simulink model "comprehensive_model_with_rocks_trial"  (R2019a)
settings: Solver=FixedStepAuto  StartTime=0.0  StopTime=15  FixedStep=0.001  RelTol=1e-3
PreLoadFcn:
  | load('tumbleweed_constants.mat')
values from neighbouring files (symbols this model uses):
  Ar = 0.785398163397    [tumbleweed_constants.mat]
  CD = 0.8    [tumbleweed_constants.mat]
  d = 0.65    [tumbleweed_constants.mat]
  g = 9.81    [tumbleweed_constants.mat]
  Ixx = 1.29    [tumbleweed_constants.mat]
  Iyy = 1.29    [tumbleweed_constants.mat]
  Izz = 1.29    [tumbleweed_constants.mat]
  m = 1    [tumbleweed_constants.mat]
  maxr = 0.45    [tumbleweed_constants.mat]
  mf = 14    [tumbleweed_constants.mat]
  minr = 0.2    [tumbleweed_constants.mat]
  mu0 = 0.02    [tumbleweed_constants.mat]
  muk = 0.5    [tumbleweed_constants.mat]
  must = 0.8    [tumbleweed_constants.mat]
  R = cylR*ones(size(Theta,1),size(Theta,2))    [d3_animate.m]    (also in tumbleweed_constants.mat = 0.5)
  rest_coeff = 0.6    [tumbleweed_constants.mat]
  rho = 1.2    [tumbleweed_constants.mat]
  ts = 0.5    [tumbleweed_constants.mat]
  v_thres = 0.0001    [tumbleweed_constants.mat]
  vmax = 0.2    [tumbleweed_constants.mat]
  YY = 50    [tumbleweed_constants.mat]
libraries: simulink x2
(part 2 of 9)

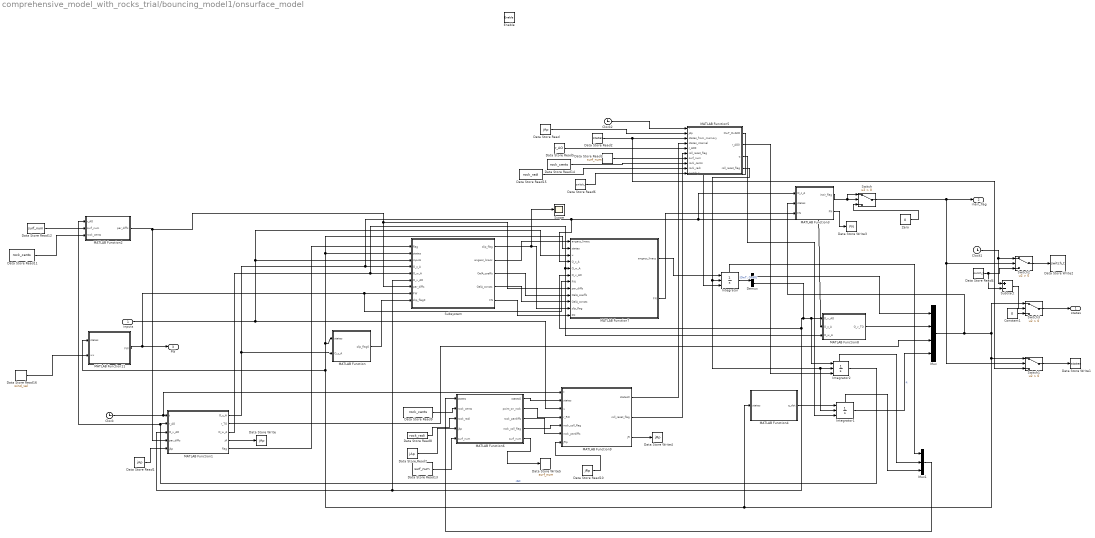
== system comprehensive_model_with_rocks_trial/bouncing_model1/onsurface_model ==
  "inputs " : Inport
  Enable : EnablePort  StatesWhenEnabling=reset
  Clock : Clock
  Clock1 : Clock
  Clock2 : Clock
  Constant1 : Constant  Value=0  VectorParams1D=off
  Data Store Read : DataStoreRead  DataStoreName=jAp
  Data Store Read1 : DataStoreRead  DataStoreName=jAp
  Data Store Read10 : DataStoreRead  DataStoreName=jRp
  Data Store Read11 : DataStoreRead  DataStoreName=rock_cents
  Data Store Read12 : DataStoreRead  DataStoreName=surf_num
  Data Store Read13 : DataStoreRead  DataStoreName=surf_num
  Data Store Read14 : DataStoreRead  DataStoreName=rock_cents
  Data Store Read15 : DataStoreRead  DataStoreName=rock_radi
  Data Store Read16 : DataStoreRead  DataStoreName=wind_vel
  Data Store Read2 : DataStoreRead  DataStoreName=states
  Data Store Read3 : DataStoreRead  DataStoreName=surf_num
  Data Store Read4 : DataStoreRead  DataStoreName=switch_t
  Data Store Read5 : DataStoreRead  DataStoreName=r_AO
  Data Store Read6 : DataStoreRead  DataStoreName=switch_t
  Data Store Read7 : DataStoreRead  DataStoreName=jAp
  Data Store Read8 : DataStoreRead  DataStoreName=rock_radi
  Data Store Read9 : DataStoreRead  DataStoreName=rock_cents
  Data Store Write : DataStoreWrite  DataStoreName=jAp
  Data Store Write1 : DataStoreWrite  DataStoreName=states
  Data Store Write2 : DataStoreWrite  DataStoreName=switch_t
  Data Store Write3 : DataStoreWrite  DataStoreName=FN
  Data Store Write4 : DataStoreWrite  DataStoreName=jRp
  Data Store Write5 : DataStoreWrite  DataStoreName=surf_num
  Demux : Demux  Outputs=[3;3]
  Integrator : Integrator  ExternalReset=level hold  InitialConditionSource=external  ShowStatePort=on
  Integrator1 : Integrator  ExternalReset=level hold  InitialConditionSource=external  ShowStatePort=on
  Integrator2 : Integrator  ExternalReset=level hold  InitialConditionSource=external  InitialCondition=[0;0;10]  ShowStatePort=on
  MATLAB Function : MATLAB Function  TreatAsAtomicUnit=on
  MATLAB Function1 : MATLAB Function  Priority=1  TreatAsAtomicUnit=on
  MATLAB Function11 : MATLAB Function  TreatAsAtomicUnit=on
  MATLAB Function2 : MATLAB Function  TreatAsAtomicUnit=on
  MATLAB Function3 : MATLAB Function  TreatAsAtomicUnit=on
  MATLAB Function4 : MATLAB Function  TreatAsAtomicUnit=on
  MATLAB Function5 : MATLAB Function  TreatAsAtomicUnit=on
  MATLAB Function6 : MATLAB Function  TreatAsAtomicUnit=on
  MATLAB Function7 : MATLAB Function  TreatAsAtomicUnit=on
  MATLAB Function8 : MATLAB Function  TreatAsAtomicUnit=on
  MATLAB Function9 : MATLAB Function  TreatAsAtomicUnit=on
  Mux : Mux  Inputs=[3;3;3;4]
  Mux1 : Mux  Inputs=[6;3;4]
  Scope : Scope
  Subsystem : Subsystem
  Subtract : Sum  Inputs=+-
  Switch{,1..3} (4 alike) : Switch  Criteria=u2 > Threshold
  Zero : Constant  Value=0  OutDataTypeStr=Inherit: Inherit via back propagation
  states : Outport
  inair_flag : Outport  Port=2  InitialOutput=1
  FW : Outport  Port=3
  wires:
  MATLAB Function2/1(par_diffs) -> MATLAB Function1/4(par_diffs), MATLAB Function7/8(par_diffs), Subsystem/7(par_diffs)
  MATLAB Function5/1(OwT_OvAO0) -> Integrator/3
  Subsystem/4(OalA_consts) -> MATLAB Function7/10(OalA_consts)
  Subsystem/3(OalA_coeffs) -> MATLAB Function7/9(OalA_coeffs)
  Subsystem/1(slip_flag) -> Scope/1, MATLAB Function7/11(slip_flag)
  Subsystem/2(angacc_linacc) -> MATLAB Function7/1("angacc_linacc ")
  MATLAB Function/1(slip_flag0) -> Subsystem/9(slip_flag0)
  "inputs "/1 -> MATLAB Function9/3(u), Subsystem/3(inputs), MATLAB Function7/3(u)
  MATLAB Function7/1(angacc_linacc) -> Integrator/1
  MATLAB Function1/5(flag) -> Subsystem/1(flag)
  Demux/2 -> Subsystem/6(O_v_AO), MATLAB Function1/3(O_v_AO), MATLAB Function7/6(O_v_AO), MATLAB Function8/1(O_v_AO), Integrator2/1
  Integrator/1 -> Demux/1  "[OwT; OvAO]"
  MATLAB Function4/1(q_dot) -> Integrator1/1
  MATLAB Function5/2(r_AO0) -> Integrator2/3
  MATLAB Function8/1(O_v_TO) -> Mux/2
  Demux/1 -> Mux/1
  Integrator2/1 -> MATLAB Function2/1(r_AO), MATLAB Function1/2(r_AO)  "rAO"
  MATLAB Function1/2(r_TO) -> Mux/3
  Integrator1/1 -> Mux/4  "q"
  MATLAB Function1/1(O_c_A) -> Subsystem/4(O_c_A), MATLAB Function8/2(O_c_A), MATLAB Function3/1(O_c_A), MATLAB Function7/4(O_c_A), MATLAB Function/2(O_c_A)
  MATLAB Function1/3(O_w_A) -> Subsystem/5(O_w_A), MATLAB Function8/3(O_w_A), MATLAB Function7/5(O_w_A)
  MATLAB Function11/1(FW) -> Subsystem/8(FW), MATLAB Function7/7(FW), FW/1
  Clock/1 -> MATLAB Function9/1(t), MATLAB Function1/1(t)
  Mux/1 -> MATLAB Function3/2(states), Subsystem/2(states), MATLAB Function7/2(states), MATLAB Function/1(states), MATLAB Function11/1(states), MATLAB Function4/1(states), Switch1/1, Switch3/1
  MATLAB Function1/4(jA) -> Data Store Write/1
  Data Store Read/1 -> MATLAB Function5/2(jAp)
  Data Store Read1/1 -> MATLAB Function1/5(jAp)
  Subsystem/5(FN) -> MATLAB Function7/12("FN ")
  MATLAB Function7/2(FN) -> MATLAB Function3/3("FN ")
  MATLAB Function3/1(inair_flag) -> Switch/1, Switch/2
  Switch/1 -> Switch2/2, Switch1/2, inair_flag/1
  Zero/1 -> Switch/3
  MATLAB Function5/3(q) -> Integrator1/3
  Switch1/1 -> Data Store Write1/1
  Switch2/1 -> Data Store Write2/1
  Data Store Read4/1 -> Subtract/2, Switch2/3
  Clock1/1 -> Subtract/1, Switch2/1
  Switch3/1 -> states/1
  Subtract/1 -> Switch3/2
  Constant1/1 -> Switch3/3
  Data Store Read5/1 -> MATLAB Function5/5("r_AO0 ")
  MATLAB Function3/2(FN) -> Data Store Write3/1
  MATLAB Function9/1(states0) -> MATLAB Function5/4(states_internal)
  Data Store Read2/1 -> Switch1/3, MATLAB Function5/3(states_from_memory)
  Data Store Read6/1 -> MATLAB Function5/10(switch_t)
  MATLAB Function6/4(rock_coll_flag) -> MATLAB Function9/5(rock_coll_flag)
  MATLAB Function6/3(rock_pardiffs) -> MATLAB Function9/6(rock_pardiffs)
  MATLAB Function6/2(point_on_rock) -> MATLAB Function9/4(r_RO)
  MATLAB Function6/1(states0) -> MATLAB Function9/2(states)
  Data Store Read7/1 -> MATLAB Function6/4(jAp)
  Data Store Read8/1 -> MATLAB Function6/3(rock_radi)
  Data Store Read9/1 -> MATLAB Function6/2(rock_cents)
  Mux1/1 -> MATLAB Function6/1(states)
  Integrator/State -> Mux1/1
  Integrator2/State -> Mux1/2
  Integrator1/State -> Mux1/3
  Data Store Read10/1 -> MATLAB Function9/7(jRp)
  MATLAB Function9/3(jR) -> Data Store Write4/1
  MATLAB Function9/2(roll_reset_flag) -> MATLAB Function5/6("roll_reset_flag ")
  MATLAB Function5/4(roll_reset_flag) -> Integrator/2, Integrator1/2, Integrator2/2
  Data Store Read3/1 -> MATLAB Function5/7(surf_num)
  Data Store Read11/1 -> MATLAB Function2/3(rock_cents)
  Data Store Read12/1 -> MATLAB Function2/2(surf_num)
  Data Store Read13/1 -> MATLAB Function6/5("surf_num ")
  Data Store Read14/1 -> MATLAB Function5/8(rock_cents)
  Data Store Read15/1 -> MATLAB Function5/9(rock_radi)
  Clock2/1 -> MATLAB Function5/1(t)
  MATLAB Function6/5(surf_num) -> Data Store Write5/1
  Data Store Read16/1 -> MATLAB Function11/2(wx)

== system comprehensive_model_with_rocks_trial/command filter based backstepper/Command filter ==
  alpha : Inport
  Demux : Demux  Commented=on  Outputs=3
  Demux1 : Demux  Commented=on  Outputs=2
  Demux2 : Demux  Commented=on  Outputs=2
  Demux3 : Demux  Commented=on  Outputs=2
  Demux4 : Demux  Outputs=3
  Gain : Gain  Gain=2
  Gain1 : Gain  Gain=2
  Gain2 : Gain  Gain=2
  Gain3 : Gain  Gain=5
  Gain4 : Gain  Gain=5
  Gain5 : Gain  Gain=5
  Integrator : Integrator
  Integrator1 : Integrator  InitialCondition=0.325
  Integrator2 : Integrator
  Integrator3 : Integrator
  Integrator4 : Integrator  InitialCondition=0.325
  Integrator5 : Integrator  InitialCondition=0.325
  Mux : Mux  Commented=on  Inputs=3
  Mux1 : Mux  Commented=on  Inputs=3
  Mux2 : Mux  Inputs=3
  Mux3 : Mux  Inputs=3
  State-Space : StateSpace  Commented=on  A=[0, 10; -2*0.8*10, -10]  B=[0;20]  C=[1,0;0,1]  D=[0;0]  InitialCondition=[0;0]
  State-Space1 : StateSpace  Commented=on  A=[0, 10; -2*0.8*10, -10]  B=[0;20]  C=[1,0;0,1]  D=[0;0]  InitialCondition=[0;0]
  State-Space2 : StateSpace  Commented=on  A=[0, 10; -2*0.8*10, -10]  B=[0;5]  C=[1,0;0,1]  D=[0;0]  InitialCondition=[0;0]
  Subtract{,1..5} (6 alike) : Sum  Inputs=+-
  wc : Outport
  wc_dot : Outport  Port=2
  wires:
  State-Space/1 -> Demux1/1
  Demux/1 -> State-Space/1
  Demux/2 -> State-Space1/1
  Demux/3 -> State-Space2/1
  State-Space1/1 -> Demux2/1
  Demux2/1 -> Mux/2
  State-Space2/1 -> Demux3/1
  Demux1/1 -> Mux/1
  Demux3/1 -> Mux/3
  Demux1/2 -> Mux1/1
  Demux2/2 -> Mux1/2
  Demux3/2 -> Mux1/3
  Mux2/1 -> wc/1
  alpha/1 -> Demux4/1
  Demux4/1 -> Subtract/1  "v1_sat"
  Gain3/1 -> Integrator/1
  Subtract/1 -> Gain/1  "v1_sat - z1"
  Subtract5/1 -> Gain5/1
  Gain/1 -> Subtract3/1
  Subtract2/1 -> Gain2/1
  Integrator2/1 -> Mux3/2, Subtract4/2, Integrator4/1
  Gain4/1 -> Integrator2/1
  Subtract1/1 -> Gain1/1
  Subtract3/1 -> Gain3/1
  Subtract4/1 -> Gain4/1
  Gain5/1 -> Integrator3/1
  Integrator/1 -> Integrator1/1, Mux3/1, Subtract3/2  "z2"
  Integrator5/1 -> Subtract2/2, Mux2/3
  Mux3/1 -> wc_dot/1
  Gain1/1 -> Subtract4/1
  Gain2/1 -> Subtract5/1
  Integrator4/1 -> Subtract1/2, Mux2/2
  Integrator3/1 -> Mux3/3, Subtract5/2, Integrator5/1
  Integrator1/1 -> Subtract/2, Mux2/1  "z1"
  Demux4/2 -> Subtract1/1
  Demux4/3 -> Subtract2/1

== system comprehensive_model_with_rocks_trial/command filter based backstepper/Subsystem ==
  v : Inport
  states : Inport  Port=2
  Add : Sum  Inputs=+-
  Add1 : Sum  Inputs=+-
  Add2 : Sum  Inputs=+-
  Demux : Demux  Outputs=3
  Derivative : Derivative  CoefficientInTFapproximation=0
  Gain : Gain  Gain=10^2
  Gain1 : Gain  Gain=2*0.1*10
  Gain2 : Gain  Gain=10^2
  Gain3 : Gain  Gain=2*0.1*10
  Gain4 : Gain  Gain=10^2
  Gain5 : Gain  Gain=2*0.1*10
  Integrator1 : Integrator  InitialCondition=d/2
  Integrator2 : Integrator  InitialCondition=d/2
  Integrator3 : Integrator  InitialCondition=d/2
  MATLAB Function : MATLAB Function  TreatAsAtomicUnit=on
  Mux : Mux  Inputs=3
  Mux1 : Mux  Inputs=3
  Saturation : Saturate  UpperLimit=vmax  LowerLimit=-vmax
  Saturation1 : Saturate  UpperLimit=vmax  LowerLimit=-vmax
  Saturation2 : Saturate  UpperLimit=maxr  LowerLimit=minr
  Saturation3 : Saturate  UpperLimit=maxr  LowerLimit=minr
  Saturation4 : Saturate  UpperLimit=vmax  LowerLimit=-vmax
  Saturation5 : Saturate  UpperLimit=maxr  LowerLimit=minr
  Subtract : Sum  Inputs=+-
  Subtract1 : Sum  Inputs=+-
  Subtract2 : Sum  Inputs=+-
  u : Outport
  u_dot : Outport  Port=2
  u_ddot : Outport  Port=3
  f3_u : Outport  Port=4
  wires:
  Saturation/1 -> Mux1/1, Gain1/1, Integrator1/1
  Demux/1 -> Saturation2/1
  Gain1/1 -> Subtract/2
  Gain/1 -> Subtract/1
  Subtract/1 -> Saturation/1
  Integrator1/1 -> Mux/1, Add/2
  Add/1 -> Gain/1
  Saturation2/1 -> Add/1
  v/1 -> Demux/1
  Saturation1/1 -> Integrator2/1, Mux1/2, Gain3/1
  Saturation3/1 -> Add1/1
  Add1/1 -> Gain2/1
  Integrator2/1 -> Add1/2, Mux/2
  Gain2/1 -> Subtract1/1
  Gain3/1 -> Subtract1/2
  Demux/2 -> Saturation3/1
  Subtract1/1 -> Saturation1/1
  Saturation4/1 -> Gain5/1, Integrator3/1
  Saturation5/1 -> Add2/1
  Add2/1 -> Gain4/1
  Integrator3/1 -> Mux1/3, Add2/2, Mux/3
  Gain4/1 -> Subtract2/1
  Gain5/1 -> Subtract2/2
  Demux/3 -> Saturation5/1
  Subtract2/1 -> Saturation4/1
  Mux1/1 -> Derivative/1, u_dot/1, MATLAB Function/2(u_dot)
  Mux/1 -> u/1, MATLAB Function/1(u)
  Derivative/1 -> MATLAB Function/3(u_ddot), u_ddot/1
  states/1 -> MATLAB Function/4(states)
  MATLAB Function/1(f3_u) -> f3_u/1

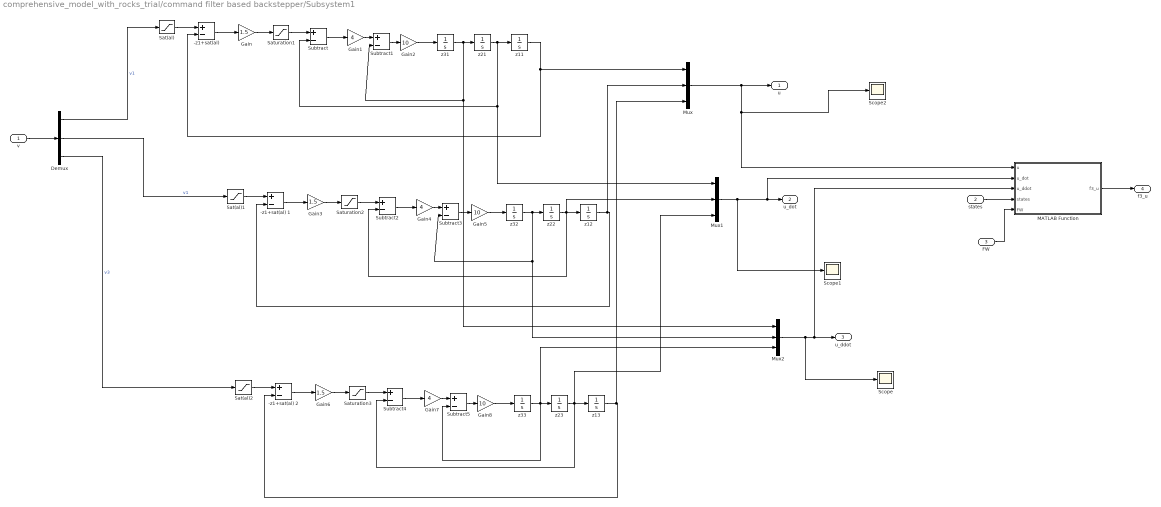
== system comprehensive_model_with_rocks_trial/command filter based backstepper/Subsystem1 ==
  v : Inport
  states : Inport  Port=2
  FW : Inport  Port=3
  "-z1+sat(al) " : Sum  Inputs=+-
  -z1+sat(al) 1 : Sum  Inputs=+-
  -z1+sat(al) 2 : Sum  Inputs=+-
  Demux : Demux  Outputs=3
  Gain : Gain  Gain=1.5
  Gain1 : Gain  Gain=4
  Gain2 : Gain  Gain=10
  Gain3 : Gain  Gain=1.5
  Gain4 : Gain  Gain=4
  Gain5 : Gain  Gain=10
  Gain6 : Gain  Gain=1.5
  Gain7 : Gain  Gain=4
  Gain8 : Gain  Gain=10
  MATLAB Function : MATLAB Function  TreatAsAtomicUnit=on
  Mux : Mux  Inputs=3
  Mux1 : Mux  Inputs=3
  Mux2 : Mux  Inputs=3
  Sat(al) : Saturate  UpperLimit=maxr  LowerLimit=minr  LinearizeAsGain=off
  Sat(al)1 : Saturate  UpperLimit=maxr  LowerLimit=minr  LinearizeAsGain=off
  Sat(al)2 : Saturate  UpperLimit=maxr  LowerLimit=minr
  Saturation1 : Saturate  UpperLimit=vmax  LowerLimit=-vmax
  Saturation2 : Saturate  UpperLimit=vmax  LowerLimit=-vmax
  Saturation3 : Saturate  UpperLimit=vmax  LowerLimit=-vmax
  Scope : Scope
  Scope1 : Scope
  Scope2 : Scope
  Subtract{,1..5} (6 alike) : Sum  Inputs=+-
  z11 : Integrator  InitialCondition=d/2
  z12 : Integrator  InitialCondition=d/2
  z13 : Integrator  InitialCondition=d/2
  z{21..23,31..33} (6 alike) : Integrator
  u : Outport
  u_dot : Outport  Port=2
  u_ddot : Outport  Port=3
  f3_u : Outport  Port=4
  wires:
  Saturation1/1 -> Subtract/1
  Subtract/1 -> Gain1/1
  Sat(al)/1 -> "-z1+sat(al) "/1
  Gain/1 -> Saturation1/1
  "-z1+sat(al) "/1 -> Gain/1
  z11/1 -> Mux/1, "-z1+sat(al) "/2
  Subtract1/1 -> Gain2/1
  z31/1 -> Mux2/1, Subtract1/2, z21/1
  Gain1/1 -> Subtract1/1
  Gain2/1 -> z31/1
  Demux/1 -> Sat(al)/1  "v1"
  v/1 -> Demux/1
  Demux/3 -> Sat(al)2/1  "v3"
  Gain5/1 -> z32/1
  Gain4/1 -> Subtract3/1
  Subtract3/1 -> Gain5/1
  z32/1 -> Mux2/2, Subtract3/2, z22/1
  Demux/2 -> Sat(al)1/1  "v1"
  z22/1 -> Mux1/2, Subtract2/2, z12/1
  z12/1 -> Mux/2, -z1+sat(al) 1/2
  -z1+sat(al) 1/1 -> Gain3/1
  Gain3/1 -> Saturation2/1
  Sat(al)1/1 -> -z1+sat(al) 1/1
  Saturation2/1 -> Subtract2/1
  Subtract2/1 -> Gain4/1
  Gain8/1 -> z33/1
  Gain7/1 -> Subtract5/1
  Subtract5/1 -> Gain8/1
  z33/1 -> Mux2/3, Subtract5/2, z23/1
  z23/1 -> Mux1/3, Subtract4/2, z13/1
  z13/1 -> Mux/3, -z1+sat(al) 2/2
  -z1+sat(al) 2/1 -> Gain6/1
  Gain6/1 -> Saturation3/1
  Sat(al)2/1 -> -z1+sat(al) 2/1
  Saturation3/1 -> Subtract4/1
  Subtract4/1 -> Gain7/1
  z21/1 -> Mux1/1, Subtract/2, z11/1
  MATLAB Function/1(f3_u) -> f3_u/1
  Mux2/1 -> Scope/1, MATLAB Function/3(u_ddot), u_ddot/1
  Mux/1 -> Scope2/1, MATLAB Function/1(u), u/1
  states/1 -> MATLAB Function/4(states)
  Mux1/1 -> Scope1/1, MATLAB Function/2(u_dot), u_dot/1
  FW/1 -> MATLAB Function/5(FW)

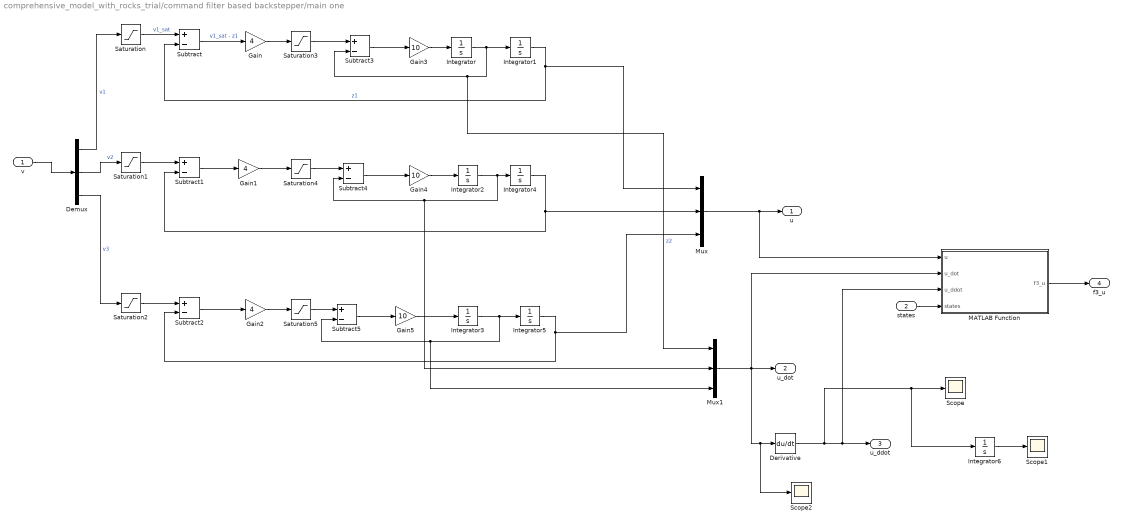
== system comprehensive_model_with_rocks_trial/command filter based backstepper/main one ==
  v : Inport
  states : Inport  Port=2
  Demux : Demux  Outputs=3
  Derivative : Derivative  CoefficientInTFapproximation=0
  Gain : Gain  Gain=4
  Gain1 : Gain  Gain=4
  Gain2 : Gain  Gain=4
  Gain3 : Gain  Gain=10
  Gain4 : Gain  Gain=10
  Gain5 : Gain  Gain=10
  Integrator{,2..3,6} (4 alike) : Integrator
  Integrator1 : Integrator  InitialCondition=d/2
  Integrator4 : Integrator  InitialCondition=d/2
  Integrator5 : Integrator  InitialCondition=d/2
  MATLAB Function : MATLAB Function  TreatAsAtomicUnit=on
  Mux : Mux  Inputs=3
  Mux1 : Mux  Inputs=3
  Saturation : Saturate  UpperLimit=maxr  LowerLimit=minr
  Saturation1 : Saturate  UpperLimit=maxr  LowerLimit=minr
  Saturation2 : Saturate  UpperLimit=maxr  LowerLimit=minr
  Saturation3 : Saturate  UpperLimit=vmax  LowerLimit=-vmax
  Saturation4 : Saturate  UpperLimit=vmax  LowerLimit=-vmax
  Saturation5 : Saturate  UpperLimit=vmax  LowerLimit=-vmax
  Scope : Scope
  Scope1 : Scope
  Scope2 : Scope
  Subtract{,1..5} (6 alike) : Sum  Inputs=+-
  u : Outport
  u_dot : Outport  Port=2
  u_ddot : Outport  Port=3
  f3_u : Outport  Port=4
  wires:
  v/1 -> Demux/1
  Demux/1 -> Saturation/1  "v1"
  Demux/2 -> Saturation1/1  "v2"
  Demux/3 -> Saturation2/1  "v3"
  Saturation/1 -> Subtract/1  "v1_sat"
  Saturation1/1 -> Subtract1/1
  Saturation2/1 -> Subtract2/1
  Subtract/1 -> Gain/1  "v1_sat - z1"
  Subtract1/1 -> Gain1/1
  Subtract2/1 -> Gain2/1
  Gain/1 -> Saturation3/1
  Gain1/1 -> Saturation4/1
  Gain2/1 -> Saturation5/1
  Saturation3/1 -> Subtract3/1
  Saturation4/1 -> Subtract4/1
  Saturation5/1 -> Subtract5/1
  Subtract3/1 -> Gain3/1
  Subtract4/1 -> Gain4/1
  Subtract5/1 -> Gain5/1
  Gain3/1 -> Integrator/1
  Integrator/1 -> Integrator1/1, Mux1/1, Subtract3/2  "z2"
  Integrator1/1 -> Subtract/2, Mux/1  "z1"
  Gain4/1 -> Integrator2/1
  Gain5/1 -> Integrator3/1
  Integrator2/1 -> Mux1/2, Subtract4/2, Integrator4/1
  Integrator4/1 -> Subtract1/2, Mux/2
  Integrator5/1 -> Subtract2/2, Mux/3
  Mux/1 -> MATLAB Function/1(u), u/1
  Integrator3/1 -> Mux1/3, Subtract5/2, Integrator5/1
  Derivative/1 -> Integrator6/1, Scope/1, MATLAB Function/3(u_ddot), u_ddot/1
  Mux1/1 -> MATLAB Function/2(u_dot), Scope2/1, Derivative/1, u_dot/1
  states/1 -> MATLAB Function/4(states)
  MATLAB Function/1(f3_u) -> f3_u/1
  Integrator6/1 -> Scope1/1

== system comprehensive_model_with_rocks_trial/command filter based backstepper1/Command filter ==
  alpha : Inport
  Demux : Demux  Commented=on  Outputs=3
  Demux1 : Demux  Commented=on  Outputs=2
  Demux2 : Demux  Commented=on  Outputs=2
  Demux3 : Demux  Commented=on  Outputs=2
  Demux4 : Demux  Outputs=3
  Gain : Gain  Gain=2
  Gain1 : Gain  Gain=2
  Gain2 : Gain  Gain=2
  Gain3 : Gain  Gain=5
  Gain4 : Gain  Gain=5
  Gain5 : Gain  Gain=5
  Integrator{,1..5} (6 alike) : Integrator
  Mux : Mux  Commented=on  Inputs=3
  Mux1 : Mux  Commented=on  Inputs=3
  Mux2 : Mux  Inputs=3
  Mux3 : Mux  Inputs=3
  State-Space : StateSpace  Commented=on  A=[0, 10; -2*0.8*10, -10]  B=[0;20]  C=[1,0;0,1]  D=[0;0]  InitialCondition=[0;0]
  State-Space1 : StateSpace  Commented=on  A=[0, 10; -2*0.8*10, -10]  B=[0;20]  C=[1,0;0,1]  D=[0;0]  InitialCondition=[0;0]
  State-Space2 : StateSpace  Commented=on  A=[0, 10; -2*0.8*10, -10]  B=[0;5]  C=[1,0;0,1]  D=[0;0]  InitialCondition=[0;0]
  Subtract{,1..5} (6 alike) : Sum  Inputs=+-
  wc : Outport
  wc_dot : Outport  Port=2
  wires:
  State-Space/1 -> Demux1/1
  Demux/1 -> State-Space/1
  Demux/2 -> State-Space1/1
  Demux/3 -> State-Space2/1
  State-Space1/1 -> Demux2/1
  Demux2/1 -> Mux/2
  State-Space2/1 -> Demux3/1
  Demux1/1 -> Mux/1
  Demux3/1 -> Mux/3
  Demux1/2 -> Mux1/1
  Demux2/2 -> Mux1/2
  Demux3/2 -> Mux1/3
  Mux2/1 -> wc/1
  alpha/1 -> Demux4/1
  Demux4/1 -> Subtract/1  "v1_sat"
  Gain3/1 -> Integrator/1
  Subtract/1 -> Gain/1  "v1_sat - z1"
  Subtract5/1 -> Gain5/1
  Gain/1 -> Subtract3/1
  Subtract2/1 -> Gain2/1
  Integrator2/1 -> Mux3/2, Subtract4/2, Integrator4/1
  Gain4/1 -> Integrator2/1
  Subtract1/1 -> Gain1/1
  Subtract3/1 -> Gain3/1
  Subtract4/1 -> Gain4/1
  Gain5/1 -> Integrator3/1
  Integrator/1 -> Integrator1/1, Mux3/1, Subtract3/2  "z2"
  Integrator5/1 -> Subtract2/2, Mux2/3
  Mux3/1 -> wc_dot/1
  Gain1/1 -> Subtract4/1
  Gain2/1 -> Subtract5/1
  Integrator4/1 -> Subtract1/2, Mux2/2
  Integrator3/1 -> Mux3/3, Subtract5/2, Integrator5/1
  Integrator1/1 -> Subtract/2, Mux2/1  "z1"
  Demux4/2 -> Subtract1/1
  Demux4/3 -> Subtract2/1

== system comprehensive_model_with_rocks_trial/command filter based backstepper1/Subsystem ==
  v : Inport
  states : Inport  Port=2
  Add : Sum  Inputs=+-
  Add1 : Sum  Inputs=+-
  Add2 : Sum  Inputs=+-
  Demux : Demux  Outputs=3
  Derivative : Derivative  CoefficientInTFapproximation=0
  Gain : Gain  Gain=10^2
  Gain1 : Gain  Gain=2*0.1*10
  Gain2 : Gain  Gain=10^2
  Gain3 : Gain  Gain=2*0.1*10
  Gain4 : Gain  Gain=10^2
  Gain5 : Gain  Gain=2*0.1*10
  Integrator1 : Integrator  InitialCondition=d/2
  Integrator2 : Integrator  InitialCondition=d/2
  Integrator3 : Integrator  InitialCondition=d/2
  MATLAB Function : MATLAB Function  TreatAsAtomicUnit=on
  Mux : Mux  Inputs=3
  Mux1 : Mux  Inputs=3
  Saturation : Saturate  UpperLimit=vmax  LowerLimit=-vmax
  Saturation1 : Saturate  UpperLimit=vmax  LowerLimit=-vmax
  Saturation2 : Saturate  UpperLimit=maxr  LowerLimit=minr
  Saturation3 : Saturate  UpperLimit=maxr  LowerLimit=minr
  Saturation4 : Saturate  UpperLimit=vmax  LowerLimit=-vmax
  Saturation5 : Saturate  UpperLimit=maxr  LowerLimit=minr
  Subtract : Sum  Inputs=+-
  Subtract1 : Sum  Inputs=+-
  Subtract2 : Sum  Inputs=+-
  u : Outport
  u_dot : Outport  Port=2
  u_ddot : Outport  Port=3
  f3_u : Outport  Port=4
  wires:
  Saturation/1 -> Mux1/1, Gain1/1, Integrator1/1
  Demux/1 -> Saturation2/1
  Gain1/1 -> Subtract/2
  Gain/1 -> Subtract/1
  Subtract/1 -> Saturation/1
  Integrator1/1 -> Mux/1, Add/2
  Add/1 -> Gain/1
  Saturation2/1 -> Add/1
  v/1 -> Demux/1
  Saturation1/1 -> Integrator2/1, Mux1/2, Gain3/1
  Saturation3/1 -> Add1/1
  Add1/1 -> Gain2/1
  Integrator2/1 -> Add1/2, Mux/2
  Gain2/1 -> Subtract1/1
  Gain3/1 -> Subtract1/2
  Demux/2 -> Saturation3/1
  Subtract1/1 -> Saturation1/1
  Saturation4/1 -> Gain5/1, Integrator3/1
  Saturation5/1 -> Add2/1
  Add2/1 -> Gain4/1
  Integrator3/1 -> Mux1/3, Add2/2, Mux/3
  Gain4/1 -> Subtract2/1
  Gain5/1 -> Subtract2/2
  Demux/3 -> Saturation5/1
  Subtract2/1 -> Saturation4/1
  Mux1/1 -> Derivative/1, u_dot/1, MATLAB Function/2(u_dot)
  Mux/1 -> u/1, MATLAB Function/1(u)
  Derivative/1 -> MATLAB Function/3(u_ddot), u_ddot/1
  states/1 -> MATLAB Function/4(states)
  MATLAB Function/1(f3_u) -> f3_u/1

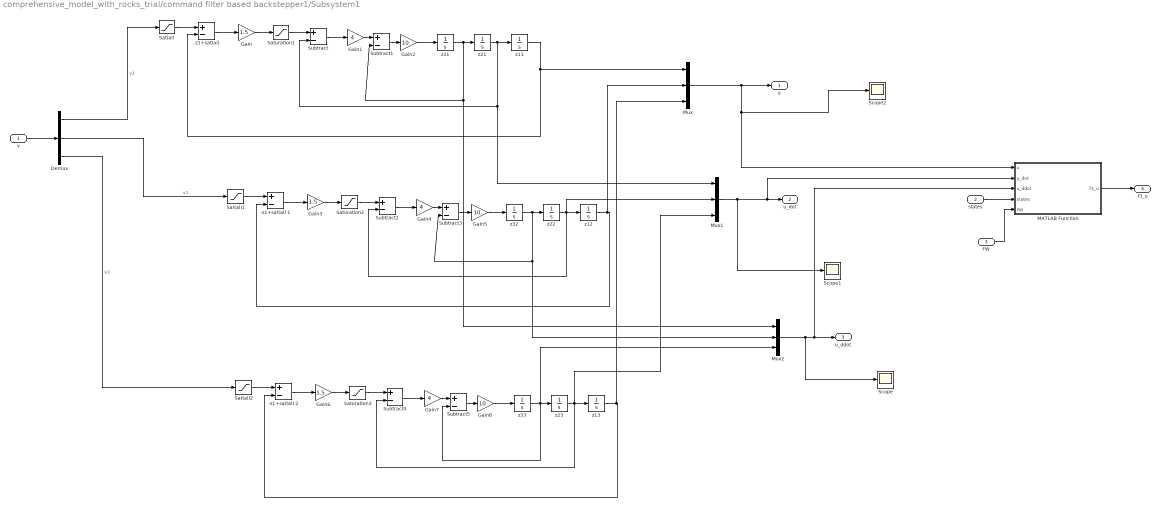
== system comprehensive_model_with_rocks_trial/command filter based backstepper1/Subsystem1 ==
  v : Inport
  states : Inport  Port=2
  FW : Inport  Port=3
  "-z1+sat(al) " : Sum  Inputs=+-
  -z1+sat(al) 1 : Sum  Inputs=+-
  -z1+sat(al) 2 : Sum  Inputs=+-
  Demux : Demux  Outputs=3
  Gain : Gain  Gain=1.5
  Gain1 : Gain  Gain=4
  Gain2 : Gain  Gain=10
  Gain3 : Gain  Gain=1.5
  Gain4 : Gain  Gain=4
  Gain5 : Gain  Gain=10
  Gain6 : Gain  Gain=1.5
  Gain7 : Gain  Gain=4
  Gain8 : Gain  Gain=10
  MATLAB Function : MATLAB Function  TreatAsAtomicUnit=on
  Mux : Mux  Inputs=3
  Mux1 : Mux  Inputs=3
  Mux2 : Mux  Inputs=3
  Sat(al) : Saturate  UpperLimit=maxr  LowerLimit=minr  LinearizeAsGain=off
  Sat(al)1 : Saturate  UpperLimit=maxr  LowerLimit=minr  LinearizeAsGain=off
  Sat(al)2 : Saturate  UpperLimit=maxr  LowerLimit=minr
  Saturation1 : Saturate  UpperLimit=vmax  LowerLimit=-vmax
  Saturation2 : Saturate  UpperLimit=vmax  LowerLimit=-vmax
  Saturation3 : Saturate  UpperLimit=vmax  LowerLimit=-vmax
  Scope : Scope
  Scope1 : Scope
  Scope2 : Scope
  Subtract{,1..5} (6 alike) : Sum  Inputs=+-
  z11 : Integrator  InitialCondition=d/2
  z12 : Integrator  InitialCondition=d/2
  z13 : Integrator  InitialCondition=d/2
  z{21..23,31..33} (6 alike) : Integrator
  u : Outport
  u_dot : Outport  Port=2
  u_ddot : Outport  Port=3
  f3_u : Outport  Port=4
  wires:
  Saturation1/1 -> Subtract/1
  Subtract/1 -> Gain1/1
  Sat(al)/1 -> "-z1+sat(al) "/1
  Gain/1 -> Saturation1/1
  "-z1+sat(al) "/1 -> Gain/1
  z11/1 -> Mux/1, "-z1+sat(al) "/2
  Subtract1/1 -> Gain2/1
  z31/1 -> Mux2/1, Subtract1/2, z21/1
  Gain1/1 -> Subtract1/1
  Gain2/1 -> z31/1
  Demux/1 -> Sat(al)/1  "v1"
  v/1 -> Demux/1
  Demux/3 -> Sat(al)2/1  "v3"
  Gain5/1 -> z32/1
  Gain4/1 -> Subtract3/1
  Subtract3/1 -> Gain5/1
  z32/1 -> Mux2/2, Subtract3/2, z22/1
  Demux/2 -> Sat(al)1/1  "v1"
  z22/1 -> Mux1/2, Subtract2/2, z12/1
  z12/1 -> Mux/2, -z1+sat(al) 1/2
  -z1+sat(al) 1/1 -> Gain3/1
  Gain3/1 -> Saturation2/1
  Sat(al)1/1 -> -z1+sat(al) 1/1
  Saturation2/1 -> Subtract2/1
  Subtract2/1 -> Gain4/1
  Gain8/1 -> z33/1
  Gain7/1 -> Subtract5/1
  Subtract5/1 -> Gain8/1
  z33/1 -> Mux2/3, Subtract5/2, z23/1
  z23/1 -> Mux1/3, Subtract4/2, z13/1
  z13/1 -> Mux/3, -z1+sat(al) 2/2
  -z1+sat(al) 2/1 -> Gain6/1
  Gain6/1 -> Saturation3/1
  Sat(al)2/1 -> -z1+sat(al) 2/1
  Saturation3/1 -> Subtract4/1
  Subtract4/1 -> Gain7/1
  z21/1 -> Mux1/1, Subtract/2, z11/1
  MATLAB Function/1(f3_u) -> f3_u/1
  Mux2/1 -> Scope/1, MATLAB Function/3(u_ddot), u_ddot/1
  Mux/1 -> Scope2/1, MATLAB Function/1(u), u/1
  states/1 -> MATLAB Function/4(states)
  Mux1/1 -> Scope1/1, MATLAB Function/2(u_dot), u_dot/1
  FW/1 -> MATLAB Function/5(FW)

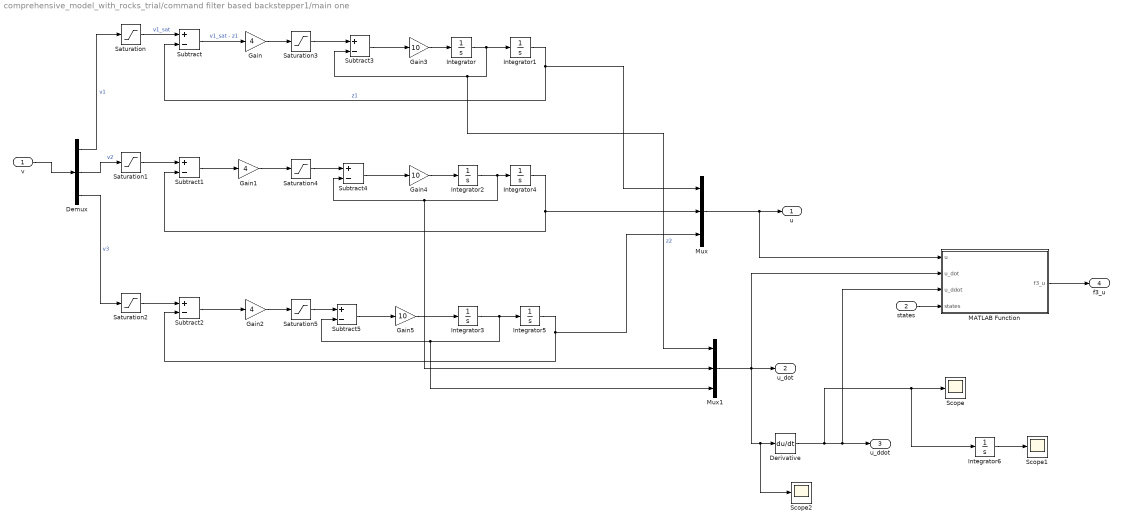
== system comprehensive_model_with_rocks_trial/command filter based backstepper1/main one ==
  v : Inport
  states : Inport  Port=2
  Demux : Demux  Outputs=3
  Derivative : Derivative  CoefficientInTFapproximation=0
  Gain : Gain  Gain=4
  Gain1 : Gain  Gain=4
  Gain2 : Gain  Gain=4
  Gain3 : Gain  Gain=10
  Gain4 : Gain  Gain=10
  Gain5 : Gain  Gain=10
  Integrator{,2..3,6} (4 alike) : Integrator
  Integrator1 : Integrator  InitialCondition=d/2
  Integrator4 : Integrator  InitialCondition=d/2
  Integrator5 : Integrator  InitialCondition=d/2
  MATLAB Function : MATLAB Function  TreatAsAtomicUnit=on
  Mux : Mux  Inputs=3
  Mux1 : Mux  Inputs=3
  Saturation : Saturate  UpperLimit=maxr  LowerLimit=minr
  Saturation1 : Saturate  UpperLimit=maxr  LowerLimit=minr
  Saturation2 : Saturate  UpperLimit=maxr  LowerLimit=minr
  Saturation3 : Saturate  UpperLimit=vmax  LowerLimit=-vmax
  Saturation4 : Saturate  UpperLimit=vmax  LowerLimit=-vmax
  Saturation5 : Saturate  UpperLimit=vmax  LowerLimit=-vmax
  Scope : Scope
  Scope1 : Scope
  Scope2 : Scope
  Subtract{,1..5} (6 alike) : Sum  Inputs=+-
  u : Outport
  u_dot : Outport  Port=2
  u_ddot : Outport  Port=3
  f3_u : Outport  Port=4
  wires:
  v/1 -> Demux/1
  Demux/1 -> Saturation/1  "v1"
  Demux/2 -> Saturation1/1  "v2"
  Demux/3 -> Saturation2/1  "v3"
  Saturation/1 -> Subtract/1  "v1_sat"
  Saturation1/1 -> Subtract1/1
  Saturation2/1 -> Subtract2/1
  Subtract/1 -> Gain/1  "v1_sat - z1"
  Subtract1/1 -> Gain1/1
  Subtract2/1 -> Gain2/1
  Gain/1 -> Saturation3/1
  Gain1/1 -> Saturation4/1
  Gain2/1 -> Saturation5/1
  Saturation3/1 -> Subtract3/1
  Saturation4/1 -> Subtract4/1
  Saturation5/1 -> Subtract5/1
  Subtract3/1 -> Gain3/1
  Subtract4/1 -> Gain4/1
  Subtract5/1 -> Gain5/1
  Gain3/1 -> Integrator/1
  Integrator/1 -> Integrator1/1, Mux1/1, Subtract3/2  "z2"
  Integrator1/1 -> Subtract/2, Mux/1  "z1"
  Gain4/1 -> Integrator2/1
  Gain5/1 -> Integrator3/1
  Integrator2/1 -> Mux1/2, Subtract4/2, Integrator4/1
  Integrator4/1 -> Subtract1/2, Mux/2
  Integrator5/1 -> Subtract2/2, Mux/3
  Mux/1 -> MATLAB Function/1(u), u/1
  Integrator3/1 -> Mux1/3, Subtract5/2, Integrator5/1
  Derivative/1 -> Integrator6/1, Scope/1, MATLAB Function/3(u_ddot), u_ddot/1
  Mux1/1 -> MATLAB Function/2(u_dot), Scope2/1, Derivative/1, u_dot/1
  states/1 -> MATLAB Function/4(states)
  MATLAB Function/1(f3_u) -> f3_u/1
  Integrator6/1 -> Scope1/1

== system comprehensive_model_with_rocks_trial/bouncing_model/onsurface_model/Subsystem ==
  flag : Inport
  states : Inport  Port=2
  inputs : Inport  Port=3
  O_c_A : Inport  Port=4
  O_w_A : Inport  Port=5
  O_v_AO : Inport  Port=6
  par_diffs : Inport  Port=7
  FW : Inport  Port=8
  slip_flag0 : Inport  Port=9
  Clock : Clock
  MATLAB Function1 : MATLAB Function  TreatAsAtomicUnit=on
  MATLAB Function2 : MATLAB Function  TreatAsAtomicUnit=on
  MATLAB Function3 : MATLAB Function  TreatAsAtomicUnit=on
  MATLAB Function6 : MATLAB Function  TreatAsAtomicUnit=on
  slip_flag : Outport
  angacc_linacc : Outport  Port=2
  OalA_coeffs : Outport  Port=3
  OalA_consts : Outport  Port=4
  FN : Outport  Port=5
  wires:
  flag/1 -> MATLAB Function2/9(flag), MATLAB Function1/1(flag)
  states/1 -> MATLAB Function6/2(states), MATLAB Function2/2(states), MATLAB Function1/2(states)
  inputs/1 -> MATLAB Function6/3(u), MATLAB Function2/3(u)
  MATLAB Function3/1(angacc_linacc) -> angacc_linacc/1, MATLAB Function6/1(angacc_linacc)
  O_v_AO/1 -> MATLAB Function1/3(O_v_AO), MATLAB Function2/6(O_v_AO)
  O_w_A/1 -> MATLAB Function6/5(O_w_A), MATLAB Function2/5(O_w_A)
  O_c_A/1 -> MATLAB Function6/4(O_c_A), MATLAB Function2/4(O_c_A)
  par_diffs/1 -> MATLAB Function1/4(par_diffs), MATLAB Function2/8(par_diffs)
  MATLAB Function2/1(A21) -> MATLAB Function3/4(A21)
  MATLAB Function2/2(A22) -> MATLAB Function3/5(A22)
  MATLAB Function2/3(B2) -> MATLAB Function3/7(B2)
  MATLAB Function1/3(B1) -> MATLAB Function3/6(B1)
  MATLAB Function1/2(A12) -> MATLAB Function3/3(A12)
  MATLAB Function1/1(A11) -> MATLAB Function3/2(A11)
  FW/1 -> MATLAB Function2/7(FW), MATLAB Function6/9(FW)
  Clock/1 -> MATLAB Function2/1(t), MATLAB Function3/1(t)
  MATLAB Function2/4(OalA_coeffs) -> OalA_coeffs/1, MATLAB Function6/6(OalA_coeffs)
  MATLAB Function2/5(OalA_consts) -> MATLAB Function6/7(OalA_consts), OalA_consts/1
  slip_flag0/1 -> MATLAB Function6/8(slip_flag0)
  MATLAB Function6/1(slip_flag) -> slip_flag/1
  MATLAB Function6/2(FN) -> FN/1

== system comprehensive_model_with_rocks_trial/bouncing_model1/onsurface_model/Subsystem ==
  flag : Inport
  states : Inport  Port=2
  inputs : Inport  Port=3
  O_c_A : Inport  Port=4
  O_w_A : Inport  Port=5
  O_v_AO : Inport  Port=6
  par_diffs : Inport  Port=7
  FW : Inport  Port=8
  slip_flag0 : Inport  Port=9
  Clock : Clock
  MATLAB Function1 : MATLAB Function  TreatAsAtomicUnit=on
  MATLAB Function2 : MATLAB Function  TreatAsAtomicUnit=on
  MATLAB Function3 : MATLAB Function  TreatAsAtomicUnit=on
  MATLAB Function6 : MATLAB Function  TreatAsAtomicUnit=on
  slip_flag : Outport
  angacc_linacc : Outport  Port=2
  OalA_coeffs : Outport  Port=3
  OalA_consts : Outport  Port=4
  FN : Outport  Port=5
  wires:
  flag/1 -> MATLAB Function2/9(flag), MATLAB Function1/1(flag)
  states/1 -> MATLAB Function6/2(states), MATLAB Function2/2(states), MATLAB Function1/2(states)
  inputs/1 -> MATLAB Function6/3(u), MATLAB Function2/3(u)
  MATLAB Function3/1(angacc_linacc) -> angacc_linacc/1, MATLAB Function6/1(angacc_linacc)
  O_v_AO/1 -> MATLAB Function1/3(O_v_AO), MATLAB Function2/6(O_v_AO)
  O_w_A/1 -> MATLAB Function6/5(O_w_A), MATLAB Function2/5(O_w_A)
  O_c_A/1 -> MATLAB Function6/4(O_c_A), MATLAB Function2/4(O_c_A)
  par_diffs/1 -> MATLAB Function1/4(par_diffs), MATLAB Function2/8(par_diffs)
  MATLAB Function2/1(A21) -> MATLAB Function3/4(A21)
  MATLAB Function2/2(A22) -> MATLAB Function3/5(A22)
  MATLAB Function2/3(B2) -> MATLAB Function3/7(B2)
  MATLAB Function1/3(B1) -> MATLAB Function3/6(B1)
  MATLAB Function1/2(A12) -> MATLAB Function3/3(A12)
  MATLAB Function1/1(A11) -> MATLAB Function3/2(A11)
  FW/1 -> MATLAB Function2/7(FW), MATLAB Function6/9(FW)
  Clock/1 -> MATLAB Function2/1(t), MATLAB Function3/1(t)
  MATLAB Function2/4(OalA_coeffs) -> OalA_coeffs/1, MATLAB Function6/6(OalA_coeffs)
  MATLAB Function2/5(OalA_consts) -> MATLAB Function6/7(OalA_consts), OalA_consts/1
  slip_flag0/1 -> MATLAB Function6/8(slip_flag0)
  MATLAB Function6/1(slip_flag) -> slip_flag/1
  MATLAB Function6/2(FN) -> FN/1

== matlab function comprehensive_model_with_rocks_trial/command filter based backstepper/MATLAB Function2 ==
  data: eta2 input; K2 input; f3_v input; f3_u input; eta2_dot output
function eta2_dot = eta2_dot_calc(eta2, K2,f3_v, f3_u)
eta2_dot = -K2*eta2 + (f3_u - f3_v);
end

== matlab function comprehensive_model_with_rocks_trial/command filter based backstepper/Subsystem/MATLAB Function ==
  data: u input; f3_u output size=3; u_dot input; u_ddot input; states input; v_thres parameter; d parameter; R parameter; mu0 parameter; mf parameter; m parameter; Izz parameter; Iyy parameter; Ixx parameter; g parameter
function f3_u = f3u_calculator(u,u_dot,u_ddot,states,v_thres, d, R, mu0, mf, m, Izz, Iyy, Ixx, g)
I_T = [Ixx,0,0;0,Iyy,0;0,0,Izz];
r_m1T = [u(1);0;0];             T_v_m1T = [u_dot(1);0;0]; T_a_m1T = [u_ddot(1);0;0];
r_m2T = [-(d - u(1));0;0];      T_v_m2T = [u_dot(1);0;0]; T_a_m2T = [u_ddot(1);0;0];
r_m3T = [0;u(2);0];             T_v_m3T = [0;u_dot(2);0]; T_a_m3T = [0;u_ddot(2);0];
r_m4T = [0;-(d - u(2));0];      T_v_m4T = [0;u_dot(2);0]; T_a_m4T = [0;u_ddot(2);0];
r_m5T = [0;0;u(3)];             T_v_m5T = [0;0;u_dot(3)]; T_a_m5T = [0;0;u_ddot(3)];
r_m6T = [0;0;-(d - u(3))];      T_v_m6T = [0;0;u_dot(3)]; T_a_m6T = [0;0;u_ddot(3)];
r_CMT = m*(r_m1T + r_m2T + r_m3T + r_m4T + r_m5T + r_m6T)/(6*m+mf);
T_v_CMT = m*(T_v_m1T + T_v_m2T + T_v_m3T + T_v_m4T + T_v_m5T + T_v_m6T)/(6*m+mf);
T_a_CMT = m*(T_a_m1T + T_a_m2T + T_a_m3T + T_a_m4T + T_a_m5T + T_a_m6T)/(6*m+mf);
r_CMTx = Vx(r_CMT);r_m1Tx = Vx(r_m1T);r_m2Tx = Vx(r_m2T);r_m3Tx = Vx(r_m3T);
r_m4Tx = Vx(r_m4T);r_m5Tx = Vx(r_m5T);r_m6Tx = Vx(r_m6T);
q0 = states(10);q1=states(11);q2=states(12);q3=states(13);
T_c_O = [q0^2 + q1^2 - q2^2 - q3^2, 2*(q1*q2 + q0*q3), 2*(q1*q3 - q0*q2);...
       2*(q1*q2 - q0*q3), q0^2 - q1^2 + q2^2 - q3^2, 2*(q2*q3 + q0*q1);...
       2*(q1*q3 + q0*q2), 2*(q2*q3 - q0*q1), q0^2 - q1^2 - q2^2 + q3^2];
O_c_T = transpose(T_c_O);  
r_PT = [0;0;-R];
r_PTx = Vx([0;0;-R]);
O_w_T = [states(1);states(2);states(3)]; O_w_Tx =Vx(O_w_T);

O_vel_TO = Vx(O_c_T*O_w_T)*[0;0;R];
u_TO = O_vel_TO(1);
v_TO = O_vel_TO(2);

murr = mu0*tanh((u_TO^2 + v_TO^2)/v_thres); 
roll_rest_coeff = [1,0,-murr*u_TO/sqrt(u_TO^2 + v_TO^2);0,1,-murr*v_TO/sqrt(u_TO^2 + v_TO^2);0,0,1];
FG = [0;0;-(mf+6*m)*g];
FR  = -murr*norm(FG)/sqrt(u_TO^2 + v_TO^2)*[u_TO; v_TO; 0];

f3_u = zeros(3,1);
Amat = I_T + (mf + 6*m)*r_CMTx*T_c_O*r_PTx*O_c_T - m*r_m1Tx*r_m1Tx - m*r_m2Tx*r_m2Tx...
       - m*r_m3Tx*r_m3Tx - m*r_m4Tx*r_m4Tx - m*r_m5Tx*r_m5Tx - m*r_m6Tx*r_m6Tx...
       - (mf + 6*m)*Vx(T_c_O*r_PT)*Vx(T_c_O*r_PT) + (mf + 6*m)*Vx(T_c_O*r_PT)*r_CMTx;
  %some mistakes here. check again 
Bvec = -cross(O_w_T,I_T*O_w_T) - m*cross(r_m1T,2*O_w_Tx*T_v_m1T + O_w_Tx*O_w_Tx*r_m1T)...
       - m*r_m2Tx*(T_a_m2T + 2*O_w_Tx*T_v_m2T + O_w_Tx*O_w_Tx*r_m2T)...
       - m*r_m3Tx*(T_a_m3T + 2*O_w_Tx*T_v_m3T + O_w_Tx*O_w_Tx*r_m3T)...
       - m*r_m4Tx*(T_a_m4T + 2*O_w_Tx*T_v_m4T + O_w_Tx*O_w_Tx*r_m4T)...
       - m*r_m5Tx*(T_a_m5T + 2*O_w_Tx*T_v_m5T + O_w_Tx*O_w_Tx*r_m5T)...
       - m*r_m6Tx*(T_a_m6T + 2*O_w_Tx*T_v_m6T + O_w_Tx*O_w_Tx*r_m6T)...
       + r_CMTx*T_c_O*FG + (mf + 6*m)*cross(T_c_O*r_PT, T_a_CMT + ...
         2*O_w_Tx*T_v_CMT + O_w_Tx*O_w_Tx*r_CMT) - T_c_O*cross(r_PT, FG) ...
         - T_c_O*cross(r_PT, FR);
f3_u = inv(Amat)*Bvec;
end

== matlab function comprehensive_model_with_rocks_trial/bouncing_model1/MATLAB Function ==
  data: states_inair input; states output; states_onsurface input; FW_inair input; FW_onsurface input; inair_flag input; FW output
function [states, FW] = merger(states_inair, states_onsurface, FW_inair, FW_onsurface, inair_flag)
if inair_flag > 0
    states = states_inair;
    FW = FW_inair;
    if norm(states) == 0
        states = states_onsurface;
        FW = FW_onsurface;
    end
else
    states = states_onsurface;
    FW = FW_onsurface;
    if norm(states) == 0
        states = states_inair;
         FW = FW_inair;
    end
end
end

== matlab function comprehensive_model_with_rocks_trial/command filter based backstepper/alpha calculator ==
  data: ref input size=3; alpha output size=3; ref_dot input; states input size=13; R parameter size=1; f1 output size=[3,3]; K1 output size=[3,3]
function [alpha, f1, K1] = alpha_calculator(ref, ref_dot, states, R)
q0 = states(10); q1 = states(11); q2 = states(12); q3 = states(13);

xc_dot = ref_dot;
xc = ref;
x = [states(7); states(8); states(9)];

K1 = 3*eye(3);

Rx = [0,R,0;-R,0,0;0,0,1];

T_c_O = [q0^2 + q1^2 - q2^2 - q3^2, 2*(q1*q2 + q0*q3), 2*(q1*q3 - q0*q2);...
2*(q1*q2 - q0*q3), q0^2 - q1^2 + q2^2 - q3^2, 2*(q2*q3 + q0*q1);...
2*(q1*q3 + q0*q2), 2*(q2*q3 - q0*q1), q0^2 - q1^2 - q2^2 + q3^2];
O_c_T = transpose(T_c_O);

f1 = Rx*O_c_T;
alpha = inv(f1)*(xc_dot - K1*(x - xc));
end

== matlab function comprehensive_model_with_rocks_trial/command filter based backstepper/main one/MATLAB Function ==
  data: u input; f3_u output size=3; u_dot input; u_ddot input; states input; v_thres parameter; d parameter; R parameter; mu0 parameter; mf parameter; m parameter; Izz parameter; Iyy parameter; Ixx parameter; g parameter
function f3_u = f3u_calculator(u,u_dot,u_ddot,states,v_thres, d, R, mu0, mf, m, Izz, Iyy, Ixx, g)
I_T = [Ixx,0,0;0,Iyy,0;0,0,Izz];
r_m1T = [u(1);0;0];             T_v_m1T = [u_dot(1);0;0]; T_a_m1T = [u_ddot(1);0;0];
r_m2T = [-(d - u(1));0;0];      T_v_m2T = [u_dot(1);0;0]; T_a_m2T = [u_ddot(1);0;0];
r_m3T = [0;u(2);0];             T_v_m3T = [0;u_dot(2);0]; T_a_m3T = [0;u_ddot(2);0];
r_m4T = [0;-(d - u(2));0];      T_v_m4T = [0;u_dot(2);0]; T_a_m4T = [0;u_ddot(2);0];
r_m5T = [0;0;u(3)];             T_v_m5T = [0;0;u_dot(3)]; T_a_m5T = [0;0;u_ddot(3)];
r_m6T = [0;0;-(d - u(3))];      T_v_m6T = [0;0;u_dot(3)]; T_a_m6T = [0;0;u_ddot(3)];
r_CMT = m*(r_m1T + r_m2T + r_m3T + r_m4T + r_m5T + r_m6T)/(6*m+mf);
T_v_CMT = m*(T_v_m1T + T_v_m2T + T_v_m3T + T_v_m4T + T_v_m5T + T_v_m6T)/(6*m+mf);
T_a_CMT = m*(T_a_m1T + T_a_m2T + T_a_m3T + T_a_m4T + T_a_m5T + T_a_m6T)/(6*m+mf);
r_CMTx = Vx(r_CMT);r_m1Tx = Vx(r_m1T);r_m2Tx = Vx(r_m2T);r_m3Tx = Vx(r_m3T);
r_m4Tx = Vx(r_m4T);r_m5Tx = Vx(r_m5T);r_m6Tx = Vx(r_m6T);
q0 = states(10);q1=states(11);q2=states(12);q3=states(13);
T_c_O = [q0^2 + q1^2 - q2^2 - q3^2, 2*(q1*q2 + q0*q3), 2*(q1*q3 - q0*q2);...
       2*(q1*q2 - q0*q3), q0^2 - q1^2 + q2^2 - q3^2, 2*(q2*q3 + q0*q1);...
       2*(q1*q3 + q0*q2), 2*(q2*q3 - q0*q1), q0^2 - q1^2 - q2^2 + q3^2];
O_c_T = transpose(T_c_O);  
r_PT = [0;0;-R];
r_PTx = Vx([0;0;-R]);
O_w_T = [states(1);states(2);states(3)]; O_w_Tx =Vx(O_w_T);

O_vel_TO = Vx(O_c_T*O_w_T)*[0;0;R];
u_TO = O_vel_TO(1);
v_TO = O_vel_TO(2);

murr = mu0*tanh((u_TO^2 + v_TO^2)/v_thres); 
roll_rest_coeff = [1,0,-murr*u_TO/sqrt(u_TO^2 + v_TO^2);0,1,-murr*v_TO/sqrt(u_TO^2 + v_TO^2);0,0,1];
FG = [0;0;-(mf+6*m)*g];
FR  = -murr*norm(FG)/sqrt(u_TO^2 + v_TO^2)*[u_TO; v_TO; 0];

f3_u = zeros(3,1);
Amat = I_T + (mf + 6*m)*r_CMTx*T_c_O*r_PTx*O_c_T - m*r_m1Tx*r_m1Tx - m*r_m2Tx*r_m2Tx...
       - m*r_m3Tx*r_m3Tx - m*r_m4Tx*r_m4Tx - m*r_m5Tx*r_m5Tx - m*r_m6Tx*r_m6Tx...
       - (mf + 6*m)*Vx(T_c_O*r_PT)*Vx(T_c_O*r_PT) + (mf + 6*m)*Vx(T_c_O*r_PT)*r_CMTx;
  %some mistakes here. check again 
Bvec = -cross(O_w_T,I_T*O_w_T) - m*cross(r_m1T,2*O_w_Tx*T_v_m1T + O_w_Tx*O_w_Tx*r_m1T)...
       - m*r_m2Tx*(T_a_m2T + 2*O_w_Tx*T_v_m2T + O_w_Tx*O_w_Tx*r_m2T)...
       - m*r_m3Tx*(T_a_m3T + 2*O_w_Tx*T_v_m3T + O_w_Tx*O_w_Tx*r_m3T)...
       - m*r_m4Tx*(T_a_m4T + 2*O_w_Tx*T_v_m4T + O_w_Tx*O_w_Tx*r_m4T)...
       - m*r_m5Tx*(T_a_m5T + 2*O_w_Tx*T_v_m5T + O_w_Tx*O_w_Tx*r_m5T)...
       - m*r_m6Tx*(T_a_m6T + 2*O_w_Tx*T_v_m6T + O_w_Tx*O_w_Tx*r_m6T)...
       + r_CMTx*T_c_O*FG + (mf + 6*m)*cross(T_c_O*r_PT, T_a_CMT + ...
         2*O_w_Tx*T_v_CMT + O_w_Tx*O_w_Tx*r_CMT) - T_c_O*cross(r_PT, FG) ...
         ;%- T_c_O*cross(r_PT, FR);
f3_u = inv(Amat)*Bvec;
end

== matlab function comprehensive_model_with_rocks_trial/command filter based backstepper/MATLAB Function1 ==
  data: eta1 input; eta1_dot output; eta2 input; alpha input; wc input; f1 input; K1 input
function eta1_dot = eta1_dot_calc(eta1, eta2, alpha, wc, f1, K1)
eta1_dot = -K1*(eta1) + f1*(wc - alpha) + f1*eta2;
end

== matlab function comprehensive_model_with_rocks_trial/command filter based backstepper/MATLAB Function ==
  data: t input; states input; rm input; v output size=3; wc input size=3; wc_dot input size=3; f1 input; ref input size=3; eta1 input; v_c input; FW input; v_thres parameter; d parameter; R parameter; mu0 parameter; mf parameter; m parameter; Izz parameter; Iyy parameter; Ixx parameter; g parameter; f3_v output size=3; K2 output size=[3,3]; fval output size=1; v_c output; M_hat output size=[3,3]; minr parameter size=1; maxr parameter size=1; vmax parameter
function [v,f3_v, K2,fval,v_c,M_hat]    = v_calculator(t, states, rm, wc, wc_dot, f1, ref, eta1, v_c,FW,v_thres, d, R, mu0, mf, m, Izz, Iyy, Ixx, g,minr, maxr, vmax)
x = [states(7);states(8);states(9)];
O_w_T = [states(1);states(2);states(3)]; 
K2 = 0.5*eye(3);
ts = 0.01;
v = zeros(3,1);
fval = 0;
if mod(t,0.1) == 0
lhs = wc_dot - K2*(O_w_T - wc) - (f1.')*(x - ref -eta1);
%FW = [0;0;0];
[v, fval] = controlsolver(ts, lhs, states, rm, FW,g, Ixx, Iyy, Izz, m, mf, mu0, R, d, v_thres, minr, maxr);


else
    v = v_c(1:3,1);
    fval = v_c(4,1);
end
v_c = [v;fval];

I_T = [Ixx,0,0;0,Iyy,0;0,0,Izz];
r_m1T = [v(1);0;0];             T_v_m1T = [rm(7);0;0]; T_a_m1T = [rm(13);0;0];
r_m2T = [-(d - v(1));0;0];      T_v_m2T = [rm(8);0;0]; T_a_m2T = [rm(14);0;0];
r_m3T = [0;v(2);0];             T_v_m3T = [0;rm(9);0]; T_a_m3T = [0;rm(15);0];
r_m4T = [0;-(d - v(2));0];      T_v_m4T = [0;rm(10);0]; T_a_m4T = [0;rm(16);0];
r_m5T = [0;0;v(3)];             T_v_m5T = [0;0;rm(11)]; T_a_m5T = [0;0;rm(17)];
r_m6T = [0;0;-(d - v(3))];      T_v_m6T = [0;0;rm(12)]; T_a_m6T = [0;0;rm(18)];
r_CMT = m*(r_m1T + r_m2T + r_m3T + r_m4T + r_m5T + r_m6T)/(6*m+mf);
T_v_CMT = m*(T_v_m1T + T_v_m2T + T_v_m3T + T_v_m4T + T_v_m5T + T_v_m6T)/(6*m+mf);
T_a_CMT = m*(T_a_m1T + T_a_m2T + T_a_m3T + T_a_m4T + T_a_m5T + T_a_m6T)/(6*m+mf);
r_CMTx = Vx(r_CMT);r_m1Tx = Vx(r_m1T);r_m2Tx = Vx(r_m2T);r_m3Tx = Vx(r_m3T);
r_m4Tx = Vx(r_m4T);r_m5Tx = Vx(r_m5T);r_m6Tx = Vx(r_m6T);
q0 = states(10);q1=states(11);q2=states(12);q3=states(13);
T_c_O = [q0^2 + q1^2 - q2^2 - q3^2, 2*(q1*q2 + q0*q3), 2*(q1*q3 - q0*q2);...
       2*(q1*q2 - q0*q3), q0^2 - q1^2 + q2^2 - q3^2, 2*(q2*q3 + q0*q1);...
       2*(q1*q3 + q0*q2), 2*(q2*q3 - q0*q1), q0^2 - q1^2 - q2^2 + q3^2];
O_c_T = transpose(T_c_O);  
r_PT = [0;0;-R];
r_PTx = Vx([0;0;-R]);
O_w_T = [states(1);states(2);states(3)]; O_w_Tx =Vx(O_w_T);

O_vel_TO = Vx(O_c_T*O_w_T)*[0;0;R];
u_TO = O_vel_TO(1);
v_TO = O_vel_TO(2);

murr = mu0*tanh((u_TO^2 + v_TO^2)/v_thres); 
roll_rest_coeff = [1,0,-murr*u_TO/sqrt(u_TO^2 + v_TO^2);0,1,-murr*v_TO/sqrt(u_TO^2 + v_TO^2);0,0,1];
FG = [0;0;-(mf+6*m)*g];
FR  = -murr*norm(FG)/sqrt(u_TO^2 + v_TO^2)*[u_TO; v_TO; 0];

Amat = I_T + (mf + 6*m)*r_CMTx*T_c_O*r_PTx*O_c_T - m*r_m1Tx*r_m1Tx - m*r_m2Tx*r_m2Tx...
       - m*r_m3Tx*r_m3Tx - m*r_m4Tx*r_m4Tx - m*r_m5Tx*r_m5Tx - m*r_m6Tx*r_m6Tx...
       - (mf + 6*m)*Vx(T_c_O*r_PT)*Vx(T_c_O*r_PT) + (mf + 6*m)*Vx(T_c_O*r_PT)*r_CMTx;
  %some mistakes here. check again 
Bvec = -cross(O_w_T,I_T*O_w_T) - m*cross(r_m1T,2*O_w_Tx*T_v_m1T + O_w_Tx*O_w_Tx*r_m1T)...
       - m*r_m2Tx*(T_a_m2T + 2*O_w_Tx*T_v_m2T + O_w_Tx*O_w_Tx*r_m2T)...
       - m*r_m3Tx*(T_a_m3T + 2*O_w_Tx*T_v_m3T + O_w_Tx*O_w_Tx*r_m3T)...
       - m*r_m4Tx*(T_a_m4T + 2*O_w_Tx*T_v_m4T + O_w_Tx*O_w_Tx*r_m4T)...
       - m*r_m5Tx*(T_a_m5T + 2*O_w_Tx*T_v_m5T + O_w_Tx*O_w_Tx*r_m5T)...
       - m*r_m6Tx*(T_a_m6T + 2*O_w_Tx*T_v_m6T + O_w_Tx*O_w_Tx*r_m6T)...
       + r_CMTx*T_c_O*FG + (mf + 6*m)*cross(T_c_O*r_PT, T_a_CMT + ...
         2*O_w_Tx*T_v_CMT + O_w_Tx*O_w_Tx*r_CMT) - T_c_O*cross(r_PT, FG) ...
        - T_c_O*cross(r_PT, FW);%- T_c_O*cross(r_PT, FR);
f3_v = Amat\Bvec;
M_hat = inv(Amat);

end

== matlab function comprehensive_model_with_rocks_trial/bouncing_model1/only_bounce/MATLAB Function ==
  data: t input; states input; u input; angacc_linacc output; FW input; inair_reset_flag input; g parameter; Ixx parameter; Iyy parameter; Izz parameter; m parameter; mf parameter
function angacc_linacc = inair_dynamics(t,states, u, FW, inair_reset_flag, g, Ixx, Iyy, Izz, m, mf)

if inair_reset_flag == 1
    disp(states);
else
    disp(states);
end
FG = [0;0;-(mf+6*m)*g];
I_T = [Ixx,0,0;0,Iyy,0;0,0,Izz]; 
r_m1T = [u(1);0;0]; T_v_m1T = [u(7);0;0]; T_a_m1T = [u(13);0;0];
r_m2T = [u(2);0;0]; T_v_m2T = [u(8);0;0]; T_a_m2T = [u(14);0;0];
r_m3T = [0;u(3);0]; T_v_m3T = [0;u(9);0]; T_a_m3T = [0;u(15);0];
r_m4T = [0;u(4);0]; T_v_m4T = [0;u(10);0]; T_a_m4T = [0;u(16);0];
r_m5T = [0;0;u(5)]; T_v_m5T = [0;0;u(11)]; T_a_m5T = [0;0;u(17)];
r_m6T = [0;0;u(6)]; T_v_m6T = [0;0;u(12)]; T_a_m6T = [0;0;u(18)];
r_CMT = m*(r_m1T + r_m2T + r_m3T + r_m4T + r_m5T + r_m6T)/(6*m+mf);
T_v_CMT = m*(T_v_m1T + T_v_m2T + T_v_m3T + T_v_m4T + T_v_m5T + T_v_m6T)/(6*m+mf);
T_a_CMT = m*(T_a_m1T + T_a_m2T + T_a_m3T + T_a_m4T + T_a_m5T + T_a_m6T)/(6*m+mf);
r_CMTx = Vx(r_CMT);r_m1Tx = Vx(r_m1T);r_m2Tx = Vx(r_m2T);r_m3Tx = Vx(r_m3T);
r_m4Tx = Vx(r_m4T);r_m5Tx = Vx(r_m5T);r_m6Tx = Vx(r_m6T);

q0 = states(10); q1 = states(11); q2 = states(12); q3 = states(13);
T_c_O = [q0^2 + q1^2 - q2^2 - q3^2, 2*(q1*q2 + q0*q3), 2*(q1*q3 - q0*q2);...
       2*(q1*q2 - q0*q3), q0^2 - q1^2 + q2^2 - q3^2, 2*(q2*q3 + q0*q1);...
       2*(q1*q3 + q0*q2), 2*(q2*q3 - q0*q1), q0^2 - q1^2 - q2^2 + q3^2];
O_c_T = T_c_O.';

O_v_TO = [states(4);states(5);states(6)];
O_w_T = [states(1);states(2);states(3)];
O_w_Tx = Vx(O_w_T);

C11 =  I_T - m*r_m1Tx*r_m1Tx - m*r_m2Tx*r_m2Tx - m*r_m3Tx*r_m3Tx - m*r_m4Tx*r_m4Tx - m*r_m5Tx*r_m5Tx - m*r_m6Tx*r_m6Tx;
C12 = (mf + 6*m)*r_CMTx*T_c_O;
C21 = -(mf + 6*m)*O_c_T*r_CMTx;
C22 = (mf + 6*m)*eye(3);
D1 = r_CMTx*T_c_O*FG - O_w_Tx*I_T*O_w_T - m*cross(r_m1T,2*O_w_Tx*T_v_m1T + O_w_Tx*O_w_Tx*r_m1T)...
       - m*r_m2Tx*(T_a_m2T + 2*O_w_Tx*T_v_m2T + O_w_Tx*O_w_Tx*r_m2T)...
       - m*r_m3Tx*(T_a_m3T + 2*O_w_Tx*T_v_m3T + O_w_Tx*O_w_Tx*r_m3T)...
       - m*r_m4Tx*(T_a_m4T + 2*O_w_Tx*T_v_m4T + O_w_Tx*O_w_Tx*r_m4T)...
       - m*r_m5Tx*(T_a_m5T + 2*O_w_Tx*T_v_m5T + O_w_Tx*O_w_Tx*r_m5T)...
       - m*r_m6Tx*(T_a_m6T + 2*O_w_Tx*T_v_m6T + O_w_Tx*O_w_Tx*r_m6T);
D2 = FG + FW - (mf + 6*m)*O_c_T*(T_a_CMT + 2*O_w_Tx*T_v_CMT + O_w_Tx*O_w_Tx*r_CMT);
C = [C11,C12;C21,C22]; D = [D1;D2];
OalT_OaTO = inv(C)*D;
O_al_T = OalT_OaTO(1:3,1);
O_a_TO = OalT_OaTO(4:6,1);
angacc_linacc = [O_al_T;O_a_TO];
end
